simulink model "mcu"  (R2025b)
settings: Solver=FixedStepDiscrete  StartTime=0.0  StopTime=10.0  FixedStep=Ts_inner  RelTol=1e-3
undefined symbols (not defined in the file): controller, imu, mahony, quadcop, Ts_batt, Ts_inner
settings Model: DataDictionary=project.sldd  Creator=Nick  LastModifiedBy=Nick
settings SolverCC: AutoInsertRateTranBlk=on
settings OptimizationCC: DefaultParameterBehavior=Inlined  EnhancedBackFolding=on  PassReuseOutputArgsAs=Individual arguments  ZeroExternalMemoryAtStartup=off  ZeroInternalMemoryAtStartup=off  OptimizeBlockOrder=speed  DifferentSizesBufferReuse=on  OptimizationCustomize=off  EfficientTunableParamExpr=on
settings DebuggingCC: ParameterTunabilityLossMsg=error
settings SFSimCC: MATLABDynamicMemAlloc=off
settings RTWCC: SystemTargetFile=ert.tlc  GenCodeOnly=on  PackageGeneratedCodeAndArtifacts=on  TemplateMakefile=ert_default_tmf  GenerateReport=on  TargetLang=C++  Description=Embedded Coder
settings CodeAppCC: ForceParamTrailComments=on  IgnoreCustomStorageClasses=off  OperatorAnnotations=on  SimulinkDataObjDesc=on  SFDataObjDesc=on  InsertBlockDesc=on
settings ERTTargetCC: RootIOFormat=Structure reference  ERTCustomFileTemplate=example_file_process.tlc  TargetLangStandard=C++11 (ISO)  GenerateSampleERTMain=on  CodeInterfacePackaging=C++ class  SubcomponentCodeInterfacePackaging=C++ class  SupportNonFinite=off

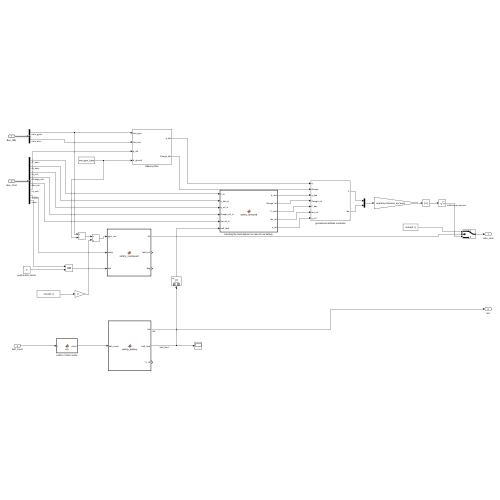
[thumbnail: Simulink's stored preview of the top-level diagram]
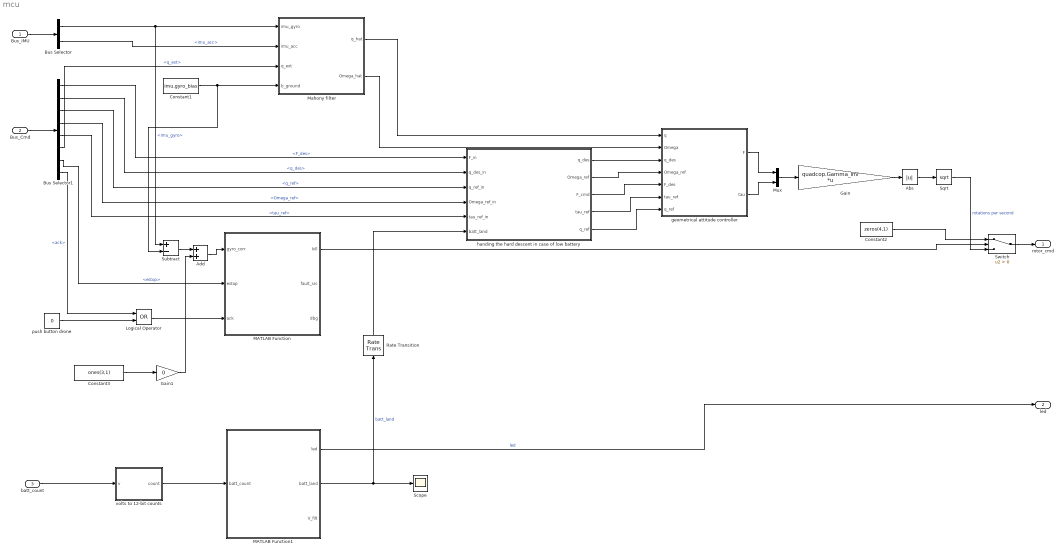
== system mcu ==
  Bus_IMU : Inport  OutDataTypeStr=Bus: Bus_IMU
  Bus_Cmd : Inport  Port=2  OutDataTypeStr=Bus: Bus_Cmd
  batt_count : Inport  Port=3
  Abs : Abs  SaturateOnIntegerOverflow=off
  Add : Sum
  Bus Selector : BusSelector  OutputSignals=imu_gyro,imu_acc
  Bus Selector1 : BusSelector  OutputSignals=F_des,q_des,q_ref,Omega_ref,tau_ref,q_ext,estop,ack
  Constant1 : Constant  Value=imu.gyro_bias
  Constant2 : Constant  Value=zeros(4,1)
  Constant3 : Constant  Value=ones(3,1)
  Gain : Gain  Gain=quadcop.Gamma_inv  Multiplication=Matrix(K*u) (u vector)
  Gain1 : Gain  Gain=0
  Logical Operator : Logic  Operator=OR  AllPortsSameDT=off  OutDataTypeStr=boolean
  MATLAB Function : MATLAB Function  TreatAsAtomicUnit=on
  MATLAB Function1 : MATLAB Function  TreatAsAtomicUnit=on  SystemSampleTime=Ts_batt
  Mahony filter : Subsystem
  Mux : Mux  Inputs=2
  Rate Transition : RateTransition  OutPortSampleTime=Ts_inner
  Scope : Scope
      settings: ActiveDisplayYMinimum=-1  ActiveDisplayYMaximum=1
  Sqrt : Sqrt
  Subtract : Sum  Inputs=+-
  Switch : Switch  Criteria=u2 > Threshold  SaturateOnIntegerOverflow=off  InputSameDT=off
  geometrical attitude controller : Subsystem
  handing the hard descent in case of low battery : MATLAB Function  TreatAsAtomicUnit=on  SystemSampleTime=Ts_inner
  push button drone : Constant  Value=0
  volts to 12-bit counts : MATLAB Function  TreatAsAtomicUnit=on
  rotor_cmd : Outport
  led : Outport  Port=2
  wires:
  Bus_IMU/1 -> Bus Selector/1
  Bus Selector/1 -> Subtract/1, Mahony filter/1(imu_gyro)  "<imu_gyro>"
  Bus Selector/2 -> Mahony filter/2(imu_acc)  "<imu_acc>"
  Bus_Cmd/1 -> Bus Selector1/1
  Bus Selector1/6 -> Mahony filter/3(q_ext)  "<q_ext>"
  Bus Selector1/4 -> handing the hard descent in case of low battery/4(Omega_ref_in)  "<Omega_ref>"
  geometrical attitude controller/1(F) -> Mux/1
  geometrical attitude controller/2(tau) -> Mux/2
  Mux/1 -> Gain/1
  Gain/1 -> Abs/1
  Mahony filter/1(q_hat) -> geometrical attitude controller/1(q)
  Mahony filter/2(Omega_hat) -> geometrical attitude controller/2(Omega)
  Bus Selector1/1 -> handing the hard descent in case of low battery/1(F_in)  "<F_des>"
  Bus Selector1/2 -> handing the hard descent in case of low battery/2(q_des_in)  "<q_des>"
  Constant1/1 -> Subtract/2, Mahony filter/4(b_ground)
  Bus Selector1/5 -> handing the hard descent in case of low battery/5(tau_ref_in)  "<tau_ref>"
  Bus Selector1/3 -> handing the hard descent in case of low battery/3(q_ref_in)  "<q_ref>"
  Abs/1 -> Sqrt/1
  Bus Selector1/7 -> MATLAB Function/2(estop)  "<estop>"
  Bus Selector1/8 -> Logical Operator/1  "<ack>"
  Logical Operator/1 -> MATLAB Function/3(ack)
  push button drone/1 -> Logical Operator/2
  MATLAB Function/1(kill) -> Switch/2
  Switch/1 -> rotor_cmd/1
  Sqrt/1 -> Switch/3  "rotations per second"
  Constant2/1 -> Switch/1
  Subtract/1 -> Add/1
  Add/1 -> MATLAB Function/1(gyro_corr)
  Constant3/1 -> Gain1/1
  Gain1/1 -> Add/2
  volts to 12-bit counts/1(count) -> MATLAB Function1/1(batt_count)
  MATLAB Function1/2(batt_land) -> Scope/1, Rate Transition/1  "batt_land"
  Rate Transition/1 -> handing the hard descent in case of low battery/6(batt_land)
  handing the hard descent in case of low battery/3(F_cmd) -> geometrical attitude controller/5(F_des)
  handing the hard descent in case of low battery/1(q_des) -> geometrical attitude controller/3(q_des)
  handing the hard descent in case of low battery/5(q_ref) -> geometrical attitude controller/7(q_ref)
  handing the hard descent in case of low battery/2(Omega_ref) -> geometrical attitude controller/4(Omega_ref)
  handing the hard descent in case of low battery/4(tau_ref) -> geometrical attitude controller/6(tau_ref)
  batt_count/1 -> volts to 12-bit counts/1(v)
  MATLAB Function1/1(led) -> led/1  "led"

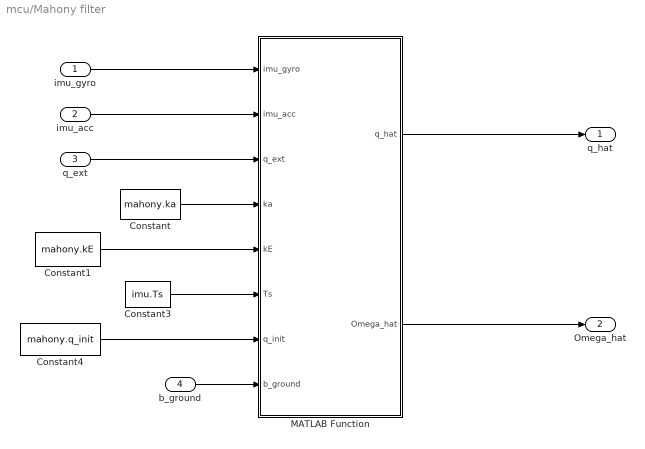
== system mcu/Mahony filter ==
  imu_gyro : Inport
  imu_acc : Inport  Port=2
  q_ext : Inport  Port=3
  b_ground : Inport  Port=4
  Constant : Constant  Value=mahony.ka
  Constant1 : Constant  Value=mahony.kE
  Constant3 : Constant  Value=imu.Ts
  Constant4 : Constant  Value=mahony.q_init
  MATLAB Function : MATLAB Function  TreatAsAtomicUnit=on
  q_hat : Outport
  Omega_hat : Outport  Port=2
  wires:
  MATLAB Function/1(q_hat) -> q_hat/1
  MATLAB Function/2(Omega_hat) -> Omega_hat/1
  imu_gyro/1 -> MATLAB Function/1(imu_gyro)
  imu_acc/1 -> MATLAB Function/2(imu_acc)
  q_ext/1 -> MATLAB Function/3(q_ext)
  Constant/1 -> MATLAB Function/4(ka)
  Constant1/1 -> MATLAB Function/5(kE)
  Constant3/1 -> MATLAB Function/6(Ts)
  Constant4/1 -> MATLAB Function/7(q_init)
  b_ground/1 -> MATLAB Function/8(b_ground)

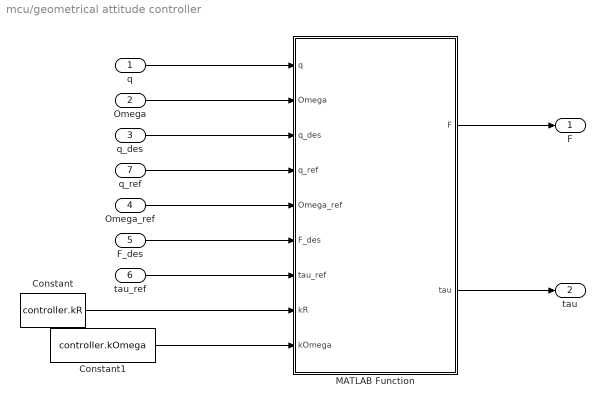
== system mcu/geometrical attitude controller ==
  q : Inport
  Omega : Inport  Port=2
  q_des : Inport  Port=3
  Omega_ref : Inport  Port=4
  F_des : Inport  Port=5
  tau_ref : Inport  Port=6
  q_ref : Inport  Port=7
  Constant : Constant  Value=controller.kR
  Constant1 : Constant  Value=controller.kOmega
  MATLAB Function : MATLAB Function  TreatAsAtomicUnit=on
  F : Outport
  tau : Outport  Port=2
  wires:
  MATLAB Function/1(F) -> F/1
  MATLAB Function/2(tau) -> tau/1
  q/1 -> MATLAB Function/1(q)
  Omega/1 -> MATLAB Function/2(Omega)
  q_des/1 -> MATLAB Function/3(q_des)
  Omega_ref/1 -> MATLAB Function/5(Omega_ref)
  F_des/1 -> MATLAB Function/6(F_des)
  tau_ref/1 -> MATLAB Function/7(tau_ref)
  Constant/1 -> MATLAB Function/8(kR)
  Constant1/1 -> MATLAB Function/9(kOmega)
  q_ref/1 -> MATLAB Function/4(q_ref)

== matlab function mcu/geometrical attitude controller/MATLAB Function ==
  data: q input; F output; Omega input; q_des input; q_ref input; Omega_ref input; F_des input; tau_ref input; kR input; kOmega input; tau output
function [F, tau] = geo_attitude_ctrl(q, Omega, q_des, q_ref, Omega_ref, F_des, tau_ref, kR, kOmega)
%#codegen
% GEO_ATTITUDE_CTRL Geometrischer Lageregler auf SO(3).
%   Lee/Leok/McClamroch (CDC 2010), 2-DOF Error-Feedback:
%       tau = tau_ff - kR*eR - kOmega*eOmega
%
%   ZWEI getrennte Referenzen (NICHT identisch!):
%     q_des : Solllage aus dem Folgeregler pos_ctrl (mit Positionsrueckfuehrung)
%             -> bestimmt den Lagefehler e_R.
%     q_ref : nominelle Solllage aus traj_gen (reine Vorsteuerung)
%             -> Frame, in dem Omega_ref definiert ist ([Om_ref]x = R_ref' R^T_ref)
%             -> Transport von Omega_ref in den aktuellen Body-Frame.
%
%
%   EIN-/AUSGAENGE:
%     q, Omega         : aktuelle Lage/Drehrate
%     q_des            : Solllage aus pos_ctrl
%     q_ref            : Solllage aus traj_gen 
%     Omega_ref        : Vorsteuer-Drehrate im Body-Frame aus traj_gen
%     F_des, tau_ff    : Vorsteuerung Schub/Moment aus traj_gen
%     kR, kOmega       : 3x3-Gains
%     F, tau           : Schubsollwert, Stellmoment

R    = quat2dcm_local(q)';      
Rdes = quat2dcm_local(q_des)';   
Rref = quat2dcm_local(q_ref)';    

% --- Lagefehler gegen die rueckgefuehrte Solllage R_des ---
S  = 0.5*(Rdes'*R - R'*Rdes);     % schiefsymmetrisch
eR = [S(3,2); S(1,3); S(2,1)];    % vee

% --- Drehratenfehler: Omega_ref aus R_ref-Frame in aktuellen Frame transportieren ---
eOmega = Omega - R'*Rref*Omega_ref;

% --- Stellgesetz ---
tau = tau_ref - kR*eR - kOmega*eOmega;
% Optional voll-geometrisch: 
% tau = tau + cross(Omega, J*Omega);

F = F_des;
end

== matlab function mcu/Mahony filter/MATLAB Function ==
  data: imu_gyro input; q_hat output; imu_acc input; q_ext input; ka input; kE input; Ts input; Omega_hat output; q_init input; b_ground input
function [q_hat, Omega_hat] = mahony_filter(imu_gyro, imu_acc, q_ext, ka, kE, Ts, q_init, b_ground)
%#codegen
% MAHONY_FILTER  Expliziter Komplementaerfilter auf SO(3), zeitdiskret.
%   Mahony/Hamel/Pflimlin (TAC 2008)). km = 0 (kein Magnetometer)
%
%     - Accel misst spezifische Kraft; im Hover [0;0;-g] -> Richtung
%       v0 = [0;0;-1]. 
%
%   EIN-/AUSGAENGE:
%     imu_gyro [rad/s] (3x1)  : gemessene Koerperdrehrate (mit Bias+Rauschen)
%     imu_acc  [m/s^2] (3x1)  : gemessene spezifische Kraft (Koerper)
%     q_ext    (4x1)          : externe Mocap-Lage 
%     ka, kE, kb (Skalar)     : Tilt-, Externreferenz-, Bias-Gain
%     Ts       [s]            : Abtastperiode 
%     q_init   (4x1)          : Startlage 
%     b_init   (3x1)          : Startbias
%     b_clamp  (Skalar)       : Maximalwert des Bias
%     q_hat    (4x1)          : geschaetzte Lage
%     Omega_hat(3x1)          : bias-korrigierte Drehrate (fuer Lageregler)
%     b_hat    (3x1)          : geschaetzter Gyro-Bias (Diagnose)
%     e_acc    (3x1)          : Innovationsterm zur Diagnose

persistent q
if isempty(q)
    q = q_init; % Startlage
end

% --- 1) Innovation (nur Richtung, Betrag traegt keine Lageinfo) ---
na = norm(imu_acc);
if na > 1e-6
    v_acc = imu_acc / na; % spezifische Kraft DCM_{be}(a -g*[0;0;-1]) in Körperkoordinaten
    v_hat = quatRotate(q, [0; 0; 1]); % geschaetzte Schwerkraftrichtung in Körperkoordinaten
    e_acc = cross(v_acc, v_hat); % Schätzfehler = Innovationsterm
else
    e_acc = [0; 0; 0]; % Freifall = unbrauchbar
end

% --- 2) Externe Mocap-Lage ---
nE = norm(q_ext);
if nE > 0.5
    qe    = q_ext / nE; % normieren da durch Quantisierung/Rauschen q_ext kein Einheitsquaternion
    q_err = quatMul(quatConj(q), qe); % Koerperinkrement, das \hat{q} -> q_ext dreht
    if q_err(1) < 0 
        q_err = -q_err; % kuerzeste Drehung, da Doppeldeckung des SO(3) durch Quaternionen
    end  
    e_ext = 2 * q_err(2:4); % Rotationsvektor (Kleinwinkel ~ Fehlerwinkel)
else
    e_ext = [0; 0; 0]; % kein gueltiges q_ext -> für Innovationsterm nur Gyro und Accel nutzen
end

% --- 3) Gewichtete Gesamt-Innovation (Koerperframe) ---
omega_mes = ka * e_acc + kE * e_ext;

% --- 5) Korrigierte Drehrate + Quaternion-Propagation ---
omega = imu_gyro - b_ground + omega_mes; % Eingang der Kinematik
theta = omega * Ts;
ang   = norm(theta);
if ang > 1e-9
    norm_theta = theta / ang;
    dq = [cos(ang/2); sin(ang/2) * norm_theta];
else
    dq = [1; 0.5 * theta]; % Kleinwinkel-Naeherung
end
q = quatMul(q, dq); % Rechtsmultiplikation = Koerperinkrement
q = q / norm(q); % auf SO(3) halten

% --- 6) Ausgaenge ---
q_hat     = q;
Omega_hat = imu_gyro - b_ground; % Bias-korrigiert
end

== matlab function mcu/MATLAB Function ==
  data: gyro_corr input double size=[3 1]; kill output boolean size=1; estop input uint8 size=1; ack input boolean size=1; fault_src output uint8 size=1; dbg output size=[3 1]; safety parameter
function [kill, fault_src, dbg] = safety_overspeed(gyro_corr, estop, ack, safety)
%#codegen
% SAFETY_OVERSPEED  Onboard-KILL-Latch
%
% Overspeed-Entprell-Latch ∪ Hard-Kill (estop==2).
% Aktion downstream: rotors_cmd = 0  (Override NACH Mixer / VOR Motor-PT1+ESC).
% KILL dominiert LAND; KILL latcht; Re-Arm NIE in der Luft.
%
% Warum eine Funktion fuer beide KILL-Quellen: Overspeed und Hard-Kill teilen
% denselben Latch, dieselbe Aktion (rotors_cmd=0) und dieselbe Re-Arm-Semantik
% (ack loescht). Eine gemeinsame Funktion haelt die Re-Arm-Bedingung an EINER
% Stelle und macht "KILL dominiert LAND" trivial. Der geregelte Soft-Land
% (estop==1) wird hier NICHT behandelt — das ist die GCS-Mode-Maschine.
%
% Eingaenge
%   gyro_corr : 3x1  bias-korrigierte Drehrate [rad/s]  (MESSUNG, nicht Schaetzer!)
%   estop : uint8  0 normal / 1 soft-land / 2 hard-kill (aus Bus_Cmd, Uplink)
%   ack : bool   Quittung, bereits ge-OR-t (Teensy-Taster-Flanke | Bus_Cmd.ack)
%   safety : struct  .omega_max [rad/s], .debounce_N (>=1), .use_norm (bool)
%
% Ausgaenge
%   kill : bool   latched -> nachgelagerter Switch zwingt rotors_cmd=0
%   fault_src : uint8  0 none / 1 overspeed / 2 hard-kill   (LED/Debug)
%   dbg : 3x1    [cnt; over_inst; ack_edge]           (verify/logging)
%
% Re-Arm (FAULT->ARMED) NUR bei:  steigende ack-Flanke  &  ~over_inst  &  estop~=2.
% Die ack-FLANKE (nicht der Pegel) verhindert, dass ein gehaltenes ack einen
% frischen Trip sofort wieder loescht oder mid-air in einen Sturz re-armt. Die
% Boden-Bedingung ("nie in der Luft") wird prozedural durch den physischen
% Teensy-Taster garantiert (Bediener hebt die Drohne auf, drueckt) — onboard
% existiert keine Pos/Vel-Schaetzung fuer ein Logik-Interlock (sitzt GCS-seitig).
% Optionaler Idle-Interlock siehe Hinweis am Dateiende.

persistent latched cnt ack_prev src
if isempty(latched)
    latched = false;
    cnt = uint16(0);
    ack_prev = false;
    src = uint8(0);
end

gw = reshape(gyro_corr, 3, 1);

% --- Overspeed-Detektor, entprellt (N aufeinanderfolgende Samples) ---
if safety.use_norm
    over_inst = sqrt(gw(1)*gw(1) + gw(2)*gw(2) + gw(3)*gw(3)) > safety.omega_max;
else
    over_inst = (abs(gw(1)) > safety.omega_max) || ...
                (abs(gw(2)) > safety.omega_max) || ...
                (abs(gw(3)) > safety.omega_max);
end

Nreq = uint16(safety.debounce_N);
if over_inst
    if cnt < Nreq
        cnt = cnt + uint16(1);
    end
else
    cnt = uint16(0);                 % ein gutes Sample setzt den Zaehler zurueck
end
over_deb = cnt >= Nreq;

% --- Hard-Kill: sofort, keine Entprellung ---
hard_kill = (estop == uint8(2));

% --- KILL setzen (latcht; Quelle nur beim ersten Setzen vermerkt) ---
if over_deb && ~latched
    latched = true;  
    src = uint8(1); % due to fast turning rates from gyro
end
if hard_kill && ~latched
    latched = true;  
    src = uint8(2);
end

% Re-Arm: steigende ack-Flanke 
ack_edge = ack && ~ack_prev;
if latched && ack_edge && ~over_inst && (estop ~= uint8(2)) % momentan kein Overspeed & kein Hard-Kill
    latched = false;
    cnt     = uint16(0);
    src     = uint8(0);
end
ack_prev = ack;

kill      = latched;
fault_src = src;
dbg       = [double(cnt); double(over_inst); double(ack_edge)];
end

% -------------------------------------------------------------------------
% OPTIONALER IDLE-INTERLOCK (nicht aktiviert):
% Will man re-arm zusaetzlich gegen "in der Luft" absichern OHNE Pos-Schaetzung,
% kann onboard ein Throttle-Idle-Proxy gefordert werden, z.B. F_ref <= F_idle:
%   ...&& (F_ref <= safety.F_rearm_idle) ...
% F_ref liegt im empfangenen Bus_Cmd vor. Das ersetzt die Boden-Schaetzung durch
% "Bediener hat heruntergeregelt", bleibt aber Heuristik (Hover braucht m*g>0).
% Bewusst NICHT verdrahtet, bis §13 das fordert.

== matlab function mcu/MATLAB Function1 ==
  data: batt_count input; led output; batt_land output boolean size=[1 1]; V_filt output double size=[1 1]; safety parameter
function [led, batt_land, V_filt] = safety_battery(batt_count, safety)
%#codegen
% safety_battery Onboard-Batterie-Monitor, 4S LiPo via PM06 V2.
%
% Kette: ADC-count --> V_batt --> V_filt --> led
%        V_filt <= V_floor --(Latch bis Reboot) --> batt_land
%
%   WARN/CRIT -> LED. Bediener im Raum sieht sie, loest MANUELL GCS-Soft-Land
%               (estop=1 => Uplink) aus, solange Marge da ist.
%   FLOOR     -> batt_land = true -> onboard BLINDER Hard-Floor-Descent 
%               (safety_landcmd.m) als Backstop, falls niemand reagiert.
% KILL (Overspeed/Hard-Kill) dominiert: rotors_cmd=0 nachgelagert sticht jeden LAND.
%
% LATCH IST PERMANENT —> KEIN Re-Arm. Zwei Gruende:
%   1) Akkuwechsel = Teensy-Reboot -> persistent wird genullt.
%   2) WICHTIGER: Im Descent faellt der Schub auf 0.98*m*g -> weniger Strom ->
%      V erholt sich UEBER den Floor. Ohne Latch wuerde batt_land deasserten,
%      das GCS-Kommando (Hover @ m*g) kaeme zurueck, Last steigt, V sackt wieder
%      -> GRENZZYKLUS Sinken<->Schweben auf fast leerem Akku. Der Latch verhindert
%      das: einmal committed -> bis zum Boden sinken.
%
% Eingaenge:
%   batt_count : ADC-Rohwert (12 bit, 0..4095). In Sim aus simulierter V-Rampe
%                (count = round((V_batt - b)/k)); auf HW analogRead(A16/Pin40).
%   safety     : struct  .batt_k .batt_b .batt_alpha .V_warn .V_crit .V_floor
%                        .V_hyst
% Ausgaenge:
%   led        : uint8  0 NORMAL / 1 WARN / 2 CRIT   (-> GPIO-Blinkmuster)
%   batt_land  : bool   latched -> safety_landcmd Hard-Floor-Override
%   V_filt     : double gefilterte Batteriespannung [V]  (dbg/logging)
%
% Hysterese: Recovery (Richtung NORMAL) braucht + V_hyst -> kein Flattern bei
% Last-Sag/Rauschen. (tau ~0.5..1 s) glaettet Sag + Rauschen UND verhindert,
% dass ein kurzer Spannungseinbruch unter Last den Floor faelschlich triggert.

persistent Vf state landed
if isempty(Vf)
    Vf     = safety.batt_k * double(batt_count) + safety.batt_b;  % init
    state  = uint8(0);
    landed = false;
end

% --- ADC -> Spannung ---
V_raw = safety.batt_k * double(batt_count) + safety.batt_b;

% --- Tiefpass: V_filt += alpha*(V_raw - V_filt) ---
Vf = Vf + safety.batt_alpha * (V_raw - Vf);
V  = Vf;

% --- 3-stufige LED mit Hysterese (Batterienzeige) ---
% NORMAL(0) -> WARN(1) -> CRIT(2); Rueckweg braucht + V_hyst.
switch state
    case uint8(0) % NORMAL
        if V <= safety.V_warn                     
            state = uint8(1); 
        end
    case uint8(1) % WARN
        if V <= safety.V_crit                 
            state = uint8(2);
        elseif V >= safety.V_warn + safety.V_hyst
            state = uint8(0); 
        end
    otherwise % CRIT (2)
        if V >= safety.V_crit + safety.V_hyst     
            state = uint8(1); 
        end
end

% --- harte Landung ---
if V <= safety.V_floor
    landed = true;
end

led       = state;
batt_land = landed;
V_filt    = V;
end

== matlab function mcu/volts to 12-bit counts ==
  data: v input; count output; safety parameter
function count = v2c(v, safety)

count = round((v - safety.batt_b)/safety.batt_k);

== matlab function mcu/handing the hard descent in case of low battery ==
  data: q_des output; Omega_ref output; F_in input; F_cmd output; tau_ref output; q_des_in input; q_ref_in input; Omega_ref_in input; tau_ref_in input; batt_land input; q_ref output; safety parameter
function [q_des, Omega_ref, F_cmd, tau_ref, q_ref] = ...
         safety_landcmd(F_in, q_des_in, q_ref_in, Omega_ref_in, tau_ref_in, ...
                        batt_land, safety)
%#codegen
% SAFETY_LANDCMD  Onboard BLINDE harte Landung
%
% Sitzt im Pfad VOR geo_attitude_ctrl. Bei batt_land = true ueberschreibt
% er den empfangenen Kommandosatz durch einen blinden Sinkflug.
% BLIND, weil onboard KEINE Pos/Vel-Schaetzung existiert. 
%
% Eingaenge: 
%   F_in         : scalar  Schub-Kommando an geo_attitude_ctrl (F = F_des)
%   q_des_in     : 4x1     Folgeregler-Lage (pos_ctrl)
%   q_ref_in     : 4x1     Vorsteuerlage (traj_gen)
%   Omega_ref_in : 3x1     Vorsteuer-Rate
%   tau_ref_in   : 3x1     Vorsteuer-Moment
%   batt_land    : bool    aus safety_battery 
%   safety       : struct  .m .g .hardfloor_thrust_frac 
% Ausgaenge an geo_attitude_ctrl.

    if batt_land
        F_cmd     = safety.hardfloor_thrust_frac * safety.m * safety.g;  % < m*g
        q_des     = [1; 0; 0; 0];     
        q_ref     = [1; 0; 0; 0];
        Omega_ref = [0; 0; 0];
        tau_ref   = [0; 0; 0];
    else
        F_cmd     = F_in;
        q_des = q_des_in;
        q_ref = q_ref_in;
        Omega_ref = Omega_ref_in;
        tau_ref = tau_ref_in;
    
    end
end
